simulink model "fork"  (R2022a)
settings: Solver=VariableStepAuto  StartTime=0.0  StopTime=6  RelTol=1e-3
libraries: simulink x1
settings Model: SnapshotBufferSize=16  SnapshotInterval=16  Creator=kasturkoul  LastModifiedBy=kasturkoul

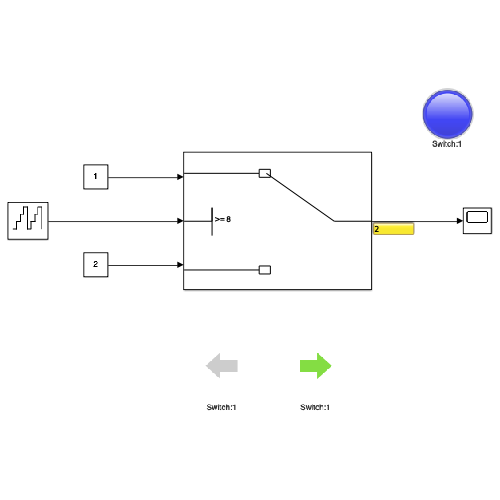
[thumbnail: Simulink's stored preview of the top-level diagram]
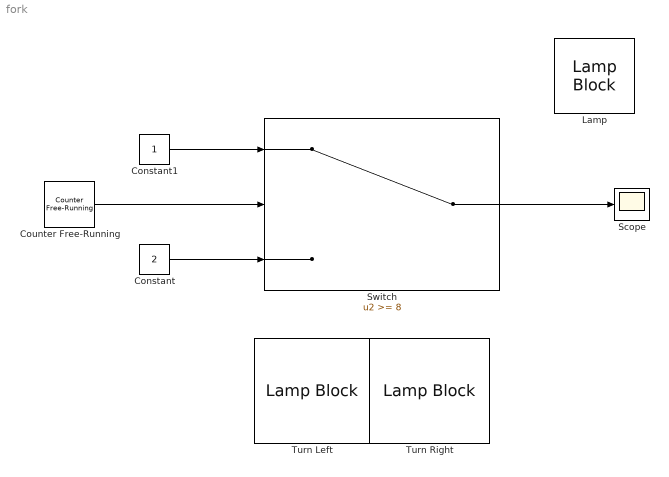
== system fork ==
  Constant : Constant  Value=2
  Constant1 : Constant
  Counter Free-Running : simulink/Sources/Counter Free-Running  NumBits=16  tsamp=-1
  Lamp : LampBlock  LabelPosition=Bottom
  Scope : Scope
  Switch : Switch  Threshold=8  SaturateOnIntegerOverflow=off  InputSameDT=off
  Turn Left : LampBlock  LabelPosition=Bottom  Icon=TurnSignalLeft
  Turn Right : LampBlock  LabelPosition=Bottom  Icon=TurnSignalRight
  wires:
  Switch/1 -> Scope/1
  Constant1/1 -> Switch/1
  Constant/1 -> Switch/3
  Counter Free-Running/1 -> Switch/2
